simulink model "Piston"  (R2023b)
settings: Solver=FixedStepAuto  StartTime=0.0  StopTime=Tsim  FixedStep=1e-3  RelTol=1e-3
values from neighbouring files (symbols this model uses):
  alpha = alpha_vec(k)    [Piston_main_nom.m]    (also in Piston_main_varyT.m = alpha_vec(j); TD_main.m = alpha_vec(i))
  Ass = ss2.a    [TD_main.m]    (also in ss_identification.m)
  Bes = 1e4*Bext    [Piston_main_nom.m]    (also in Piston_main_varyT.m; TD_main.m)
  Bext = SF^2.5*Bext_ref    (= 2000)    [Hydrodynamic_parameters_scaling.m]
  Bss = ss2.b    [TD_main.m]    (also in ss_identification.m)
  Css = ss2.c    [TD_main.m]    (also in ss_identification.m)
  d = SF*d_ref    (= 4.7)    [Hydrodynamic_parameters_scaling.m]
  Fs1data = table2array(readtable('..\Fs1data.xls'))    [Piston.m]    (also in data_grids.m)
  Fw = compute_Fw(ss_type, H, T, omega, gamma, t)    [Piston_main_nom.m]    (also in Piston_main_varyT.m; TD_main.m = Fw + gamma(i)*sqrt(2*(omega(2)-omega(1))*Som(i))*sin(omega(i; compute_Fw.m = Fw + gamma(i)*sqrt(2*(omega(2)-omega(1))*Som(i))*sin(omega(i)
  Kb = rho*g*pi*r^2    (= 198397.46656)    [Hydrodynamic_parameters_scaling.m]
  Kes = 1e0*Kb    [Piston_main_nom.m]    (also in Piston_main_varyT.m; TD_main.m)
  M = SF^3*M_ref    [Hydrodynamic_parameters_scaling.m]
  V1data = table2array(readtable('..\V1data.xls'))    [Piston.m]    (also in data_grids.m)
  V1max = 50e3    (= 50000)    [Piston.m]    (also in data_grids.m = max(V1data))
  V2max = 50e3    (= 50000)    [Piston.m]    (also in data_grids.m = max(V2data))
  Vmax = 20    [Piston_main_nom.m]    (also in Piston_main_varyT.m; TD_main.m)
  z1data = table2array(readtable('..\z1data.xls'))    [Piston.m]    (also in data_grids.m)
settings Model: SimulationMode=accelerator  Creator=massi  LastModifiedBy=massi

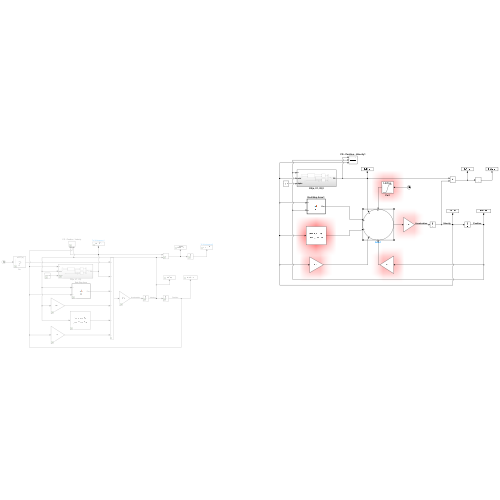
[thumbnail: Simulink's stored preview of the top-level diagram]
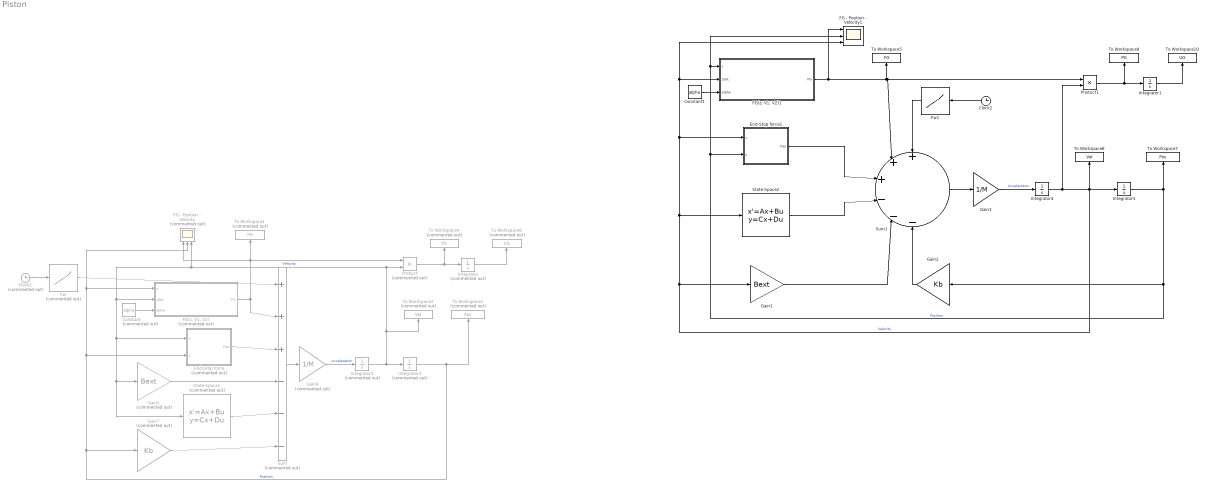
== system Piston ==
  Clock1 : Clock  Commented=on
  Clock2 : Clock
  Constant : Constant  Commented=on  Value=alpha
  Constant1 : Constant  Value=alpha
  End-Stop force : MATLAB Function  Commented=on  TreatAsAtomicUnit=on
  End-Stop force1 : MATLAB Function  TreatAsAtomicUnit=on
  FG - Position - Velocity : Scope  Commented=on  NumInputPorts=3
  FG - Position - Velocity1 : Scope  NumInputPorts=3
  "FG(z, V1, V2)" : Subsystem  Commented=on
  "FG(z, V1, V2)1" : Subsystem
  Fw : Lookup_n-D  Commented=on  NumberOfTableDimensions=1  BreakpointsForDimension1=t  Table=Fw  InternalRulePriority=Speed  RndMeth=Simplest
  Fw1 : Lookup_n-D  NumberOfTableDimensions=1  BreakpointsForDimension1=t  Table=Fw  InternalRulePriority=Speed  RndMeth=Simplest
  Gain1 : Gain  Gain=Bext
  Gain2 : Gain  Gain=Kb
  Gain3 : Gain  Gain=1/M
  Gain5 : Gain  Commented=on  Gain=Bext
  Gain7 : Gain  Commented=on  Gain=Kb
  Gain9 : Gain  Commented=on  Gain=1/M
  Integrator : Integrator  Commented=on
  Integrator1 : Integrator
  Integrator2 : Integrator  Commented=on
  Integrator3 : Integrator  Commented=on
  Integrator4 : Integrator
  Integrator5 : Integrator
  Product : Product  Commented=on
  Product1 : Product
  State-Space1 : StateSpace  Commented=on  A=Ass  B=Bss  C=Css  D=0  InitialCondition=0
  State-Space2 : StateSpace  A=Ass  B=Bss  C=Css  D=0  InitialCondition=0
  Sum : Sum  Commented=on  Inputs=+|+|+|-|-|-
  Sum1 : Sum  Inputs=+|+|+|-|-|-
  To Workspace1 : ToWorkspace  Commented=on  VariableName=FG  SaveFormat=Timeseries  SampleTime=-1
  To Workspace10 : ToWorkspace  VariableName=UG  SaveFormat=Timeseries  SampleTime=-1
  To Workspace2 : ToWorkspace  Commented=on  VariableName=Pos  SaveFormat=Timeseries  SampleTime=-1
  To Workspace3 : ToWorkspace  Commented=on  VariableName=Vel  SaveFormat=Timeseries  SampleTime=-1
  To Workspace4 : ToWorkspace  Commented=on  VariableName=PG  SaveFormat=Timeseries  SampleTime=-1
  To Workspace5 : ToWorkspace  VariableName=FG  SaveFormat=Timeseries  SampleTime=-1
  To Workspace6 : ToWorkspace  Commented=on  VariableName=UG  SaveFormat=Timeseries  SampleTime=-1
  To Workspace7 : ToWorkspace  VariableName=Pos  SaveFormat=Timeseries  SampleTime=-1
  To Workspace8 : ToWorkspace  VariableName=Vel  SaveFormat=Timeseries  SampleTime=-1
  To Workspace9 : ToWorkspace  VariableName=PG  SaveFormat=Timeseries  SampleTime=-1
  wires:
  Clock1/1 -> Fw/1
  Fw/1 -> Sum/1
  "FG(z, V1, V2)"/1(FG) -> Sum/2, Product/1, To Workspace1/1, FG - Position - Velocity/1
  Constant/1 -> "FG(z, V1, V2)"/3(alpha)
  End-Stop force/1(Fes) -> Sum/3
  Sum/1 -> Gain9/1
  Gain9/1 -> Integrator2/1  "Acceleration"
  Integrator2/1 -> Product/2, FG - Position - Velocity/3, State-Space1/1, Gain5/1, End-Stop force/1(v), "FG(z, V1, V2)"/2(zdot), To Workspace3/1, Integrator3/1  "Velocity"
  Integrator3/1 -> To Workspace2/1, Gain7/1, End-Stop force/2(z), "FG(z, V1, V2)"/1(z), FG - Position - Velocity/2  "Position"
  Product/1 -> To Workspace4/1, Integrator/1
  Integrator/1 -> To Workspace6/1
  Gain7/1 -> Sum/6
  State-Space1/1 -> Sum/5
  Gain5/1 -> Sum/4
  Gain2/1 -> Sum1/6
  "FG(z, V1, V2)1"/1(FG) -> Sum1/2, Product1/1, To Workspace5/1, FG - Position - Velocity1/1
  Constant1/1 -> "FG(z, V1, V2)1"/3(alpha)
  Integrator1/1 -> To Workspace10/1
  Product1/1 -> Integrator1/1, To Workspace9/1
  Fw1/1 -> Sum1/1
  Sum1/1 -> Gain3/1
  Gain3/1 -> Integrator4/1  "Acceleration"
  Clock2/1 -> Fw1/1
  Integrator4/1 -> To Workspace8/1, Integrator5/1, FG - Position - Velocity1/3, "FG(z, V1, V2)1"/2(zdot), End-Stop force1/1(v), State-Space2/1, Gain1/1, Product1/2  "Velocity"
  End-Stop force1/1(Fes) -> Sum1/3
  Gain1/1 -> Sum1/5
  State-Space2/1 -> Sum1/4
  Integrator5/1 -> Gain2/1, FG - Position - Velocity1/2, "FG(z, V1, V2)1"/1(z), End-Stop force1/2(z), To Workspace7/1  "Position"

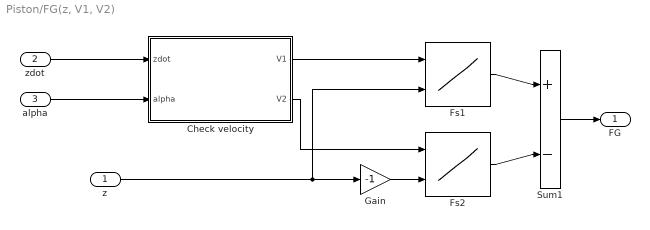
== system Piston/FG(z, V1, V2) ==
  z : Inport
  zdot : Inport  Port=2
  alpha : Inport  Port=3
  Check velocity : MATLAB Function  TreatAsAtomicUnit=on
  Fs1 : Lookup_n-D  BreakpointsForDimension1=V1data  BreakpointsForDimension2=z1data  Table=Fs1data  DiagnosticForOutOfRangeInput=Error  InternalRulePriority=Speed  RndMeth=Simplest
      settings: InputPortMap=u0,u1
  Fs2 : Lookup_n-D  BreakpointsForDimension1=V1data  BreakpointsForDimension2=z1data  Table=Fs1data  DiagnosticForOutOfRangeInput=Error  InternalRulePriority=Speed  RndMeth=Simplest
      settings: InputPortMap=u0,u1
  Gain : Gain  Gain=-1
  Sum1 : Sum  Inputs=+|-
  FG : Outport
  wires:
  Fs1/1 -> Sum1/1
  alpha/1 -> Check velocity/2(alpha)
  Fs2/1 -> Sum1/2
  Check velocity/2(V2) -> Fs2/1
  Check velocity/1(V1) -> Fs1/1
  Sum1/1 -> FG/1
  z/1 -> Gain/1, Fs1/2
  Gain/1 -> Fs2/2
  zdot/1 -> Check velocity/1(zdot)

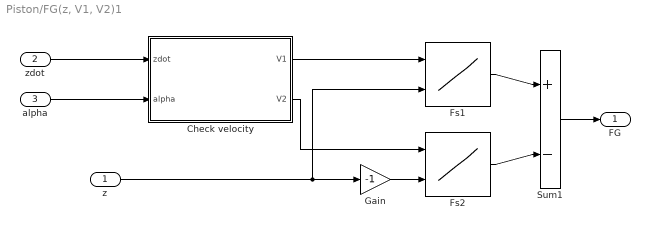
== system Piston/FG(z, V1, V2)1 ==
  z : Inport
  zdot : Inport  Port=2
  alpha : Inport  Port=3
  Check velocity : MATLAB Function  TreatAsAtomicUnit=on
  Fs1 : Lookup_n-D  BreakpointsForDimension1=V1data  BreakpointsForDimension2=z1data  Table=Fs1data  DiagnosticForOutOfRangeInput=Error  InternalRulePriority=Speed  RndMeth=Simplest
      settings: InputPortMap=u0,u1
  Fs2 : Lookup_n-D  BreakpointsForDimension1=V1data  BreakpointsForDimension2=z1data  Table=Fs1data  DiagnosticForOutOfRangeInput=Error  InternalRulePriority=Speed  RndMeth=Simplest
      settings: InputPortMap=u0,u1
  Gain : Gain  Gain=-1
  Sum1 : Sum  Inputs=+|-
  FG : Outport
  wires:
  Fs1/1 -> Sum1/1
  alpha/1 -> Check velocity/2(alpha)
  Fs2/1 -> Sum1/2
  Check velocity/2(V2) -> Fs2/1
  Check velocity/1(V1) -> Fs1/1
  Sum1/1 -> FG/1
  z/1 -> Gain/1, Fs1/2
  Gain/1 -> Fs2/2
  zdot/1 -> Check velocity/1(zdot)

== matlab function Piston/FG(z, V1, V2)/Check velocity ==
  data: zdot input; V1 output; alpha input; V2 output; V1max parameter; V2max parameter
function [V1,V2] = check_zdot(zdot, alpha,V1max, V2max)
    
    if zdot >= 1e-3
        V1 = 0;
        V2 = alpha * V2max;
    elseif zdot < -1e-3
        V2 = 0;
        V1 = alpha * V1max;
    else 
        V1 = 0;
        V2 = 0;
    end

end

== matlab function Piston/End-Stop force1 ==
  data: v input; Fes output; z input; d parameter; Kes parameter; Bes parameter; Vmax parameter
function Fes = fcn(v,z,d,Kes, Bes, Vmax)

if abs(z)<d
    Fes = 0;
elseif z>d
    Fes = -Kes*(z-d)-Bes*v;
else
    Fes = -Kes*(z+d)-Bes*v;
end

if abs(v)>Vmax
    Fes = Fes -Bes*v;
end

== matlab function Piston/End-Stop force ==
  data: v input; Fes output; z input; d parameter; Kes parameter; Bes parameter; Vmax parameter
function Fes = fcn(v,z,d,Kes, Bes, Vmax)

if abs(z)<d
    Fes = 0;
elseif z>d
    Fes = -Kes*(z-d)-Bes*v;
else
    Fes = -Kes*(z+d)-Bes*v;
end

if abs(v)>Vmax
    Fes = Fes -Bes*v;
end

== matlab function Piston/FG(z, V1, V2)1/Check velocity ==
  data: zdot input; V1 output; alpha input; V2 output; V1max parameter; V2max parameter
function [V1,V2] = check_zdot(zdot, alpha,V1max, V2max)
    
    if zdot >= 1e-3
        V1 = 0;
        V2 = alpha * V2max;
    elseif zdot < -1e-3
        V2 = 0;
        V1 = alpha * V1max;
    else 
        V1 = 0;
        V2 = 0;
    end

end
